simulink library "csm"  (Simulink 8.1)
settings: Solver=ode1  StartTime=0.0  StopTime=Inf  FixedStep=0.001  RelTol=1e-3
PostLoadFcn:
  | , if any(exist('dsrtsu_mdlpostloadfcn', 'file') == [2, 3, 6]), try dsrtsu_mdlpostloadfcn('Execute', bdroot); catch fprintf('Error in PostLoadFcn (dsrtsu_mdlpostloadfcn) for model "%s":\n %s\n', bdroot, lasterr); end, end,
libraries: simulink x1, hcu_lib x1
settings Model: DSRTSU_INTERNAL_RTI_VER=450  DSRTSU_INTERNAL_RTI_TYPE=rti1401  RTICANMMDATA=struct('GeneralSetupData',struct('modelroot','D:\Projects\ELN150201\Repositories\Taiwan\trunk\AdasDragon\software\sw_development\arch\app\jud','generalsettings',struct('filesettings',struct('destfolder',struct('Name','RTICANMM_FILES','Check',1),'buildfolder',struct('Name','.','Check',1),'AbsDestfolder',struct('Name','D:\Projects\ELN150201\Repositories\Taiwan\trunk\AdasDragon\software\sw_development\arch\app\jud\RTICANMM_FILES'),'AbsBuildfolder',struct('Name','D:\Projects\ELN150201\Repositories\Taiwan\trunk\AdasDragon\software\sw_development\arch\app\jud'))),'options',struct('addpaths',1,'rmpaths',1,'addtrcexclusion',logical(1),'cannavigator',struct('checkmonitoring',0),'show_usrtrc',0,'use_usrtrc',0),'advanced',struct('options',[1 1 1 1 1 1 1 1 1 1 1 1 1 1 1 1 1 1 1 1 1 1 1 1 1 1 1 1 1 1 1 1 1 1 1 1 1 1 1 1 1 1 1 1 1 1 1 1 1 1 1 1 1 1 1 1 1 1 1 1 1 1 1 1 1 1 1 1 1 1 1 1 1 1 1 1 1 1 1 1 1 1 1 1 1 1 1 1 1 1 1 1 1 1 1 1 1 1 1 1]),'MPSetup',{{}},'modelname','csm','block','csm'))  DSRTSU_INTERNAL_RTIFPGA=40  Creator=AT015411  LastModifiedBy=AT015086

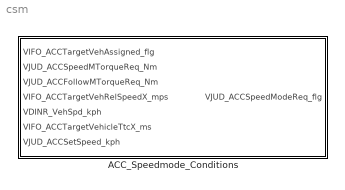
== system csm ==
  ACC_Speedmode_Conditions : Subsystem

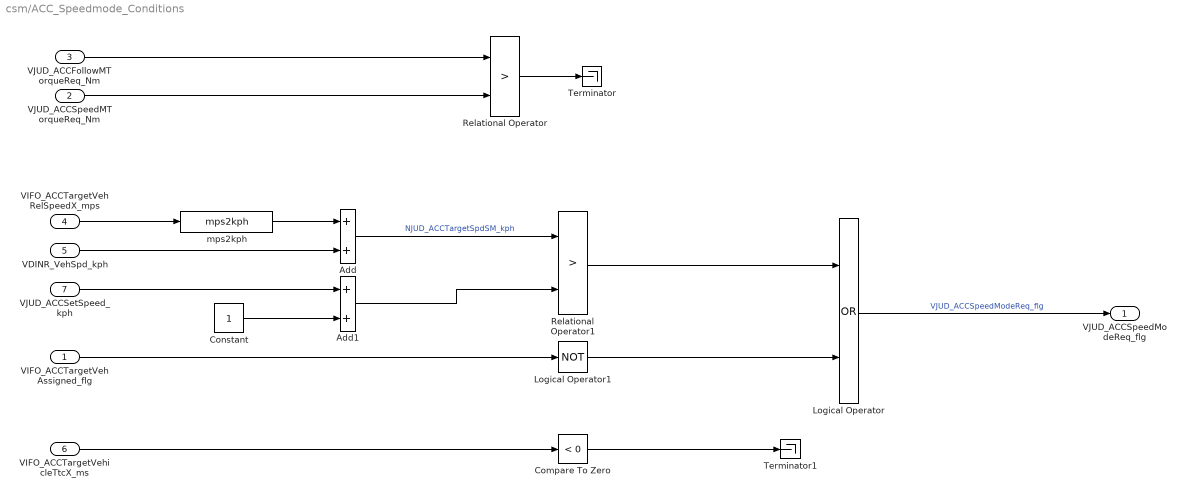
== system csm/ACC_Speedmode_Conditions ==
  VIFO_ACCTargetVehAssigned_flg : Inport
  VJUD_ACCSpeedMTorqueReq_Nm : Inport  Port=2
  VJUD_ACCFollowMTorqueReq_Nm : Inport  Port=3
  VIFO_ACCTargetVehRelSpeedX_mps : Inport  Port=4
  VDINR_VehSpd_kph : Inport  Port=5
  VIFO_ACCTargetVehicleTtcX_ms : Inport  Port=6
  VJUD_ACCSetSpeed_kph : Inport  Port=7
  Add : Sum
  Add1 : Sum
  Compare To Zero : simulink/Logic and Bit Operations/Compare To Zero  relop=<  OutDataTypeStr=boolean
  Constant : Constant
  Logical Operator : Logic  Operator=OR  AllPortsSameDT=off  OutDataTypeStr=boolean
  Logical Operator1 : Logic  Operator=NOT  AllPortsSameDT=off  OutDataTypeStr=boolean
  Relational Operator : RelationalOperator  Operator=>  OutDataTypeStr=boolean
  Relational Operator1 : RelationalOperator  Operator=>  OutDataTypeStr=boolean
  Terminator : Terminator
  Terminator1 : Terminator
  mps2kph : hcu_lib/mps2kph
  VJUD_ACCSpeedModeReq_flg : Outport
  wires:
  Relational Operator1/1 -> Logical Operator/1
  Add/1 -> Relational Operator1/1  "NJUD_ACCTargetSpdSM_kph"
  mps2kph/1 -> Add/1
  VIFO_ACCTargetVehRelSpeedX_mps/1 -> mps2kph/1
  VDINR_VehSpd_kph/1 -> Add/2
  VJUD_ACCSetSpeed_kph/1 -> Add1/1
  Relational Operator/1 -> Terminator/1
  Logical Operator/1 -> VJUD_ACCSpeedModeReq_flg/1  "VJUD_ACCSpeedModeReq_flg"
  VJUD_ACCFollowMTorqueReq_Nm/1 -> Relational Operator/1
  VJUD_ACCSpeedMTorqueReq_Nm/1 -> Relational Operator/2
  VIFO_ACCTargetVehAssigned_flg/1 -> Logical Operator1/1
  Logical Operator1/1 -> Logical Operator/2
  VIFO_ACCTargetVehicleTtcX_ms/1 -> Compare To Zero/1
  Compare To Zero/1 -> Terminator1/1
  Constant/1 -> Add1/2
  Add1/1 -> Relational Operator1/2
